simulink model "OptimalTracking_F16_Simulink"  (R2020b)
settings: Solver=VariableStepAuto  StartTime=0.0  StopTime=30  RelTol=1e-3
values from neighbouring files (symbols this model uses):
  A = [0 0 1 ... (first row only)    [OptimalTracking_F16.m]
  B = [0 ... (first row only)    [OptimalTracking_F16.m]
  C = [1 0 0]    [OptimalTracking_F16.m]
  G1 = -inv(C*inv(A-B*K1)*B)    [OptimalTracking_F16.m]
  G2 = -inv(C*inv(A-B*K2)*B)    [OptimalTracking_F16.m]
  G3 = -inv(C*inv(A-B*K3)*B)    [OptimalTracking_F16.m]
  G4 = -inv(C*inv(A-B*K4)*B)    [OptimalTracking_F16.m]
  G_f = -inv(C*inv(A-B*K_f)*B)    [OptimalTracking_F16.m]
  G_s = -inv(C*inv(A-B*K_s)*B)    [OptimalTracking_F16.m]
  G_t = -inv(C*inv(A-B*K_t)*B)    [OptimalTracking_F16.m]
  K1 = place(A,B,PO)    [OptimalTracking_F16.m]
  K2 = lqr(A,B,Q1,R1)    [OptimalTracking_F16.m]
  K3 = lqr(A,B,Q2,R2)    [OptimalTracking_F16.m]
  K4 = lqr(A,B,Q3,R3)    [OptimalTracking_F16.m]
  K_f = lqr(A,B,Q_u,r1)    [OptimalTracking_F16.m]
  K_s = lqr(A,B,Q_u,r2)    [OptimalTracking_F16.m]
  K_t = lqr(A,B,Q_u,r3)    [OptimalTracking_F16.m]
  u_opt = double(u_opt)    [Zermelo.m]
libraries: simulink_extras x6
settings Model: Creator=DELL  LastModifiedBy=DELL

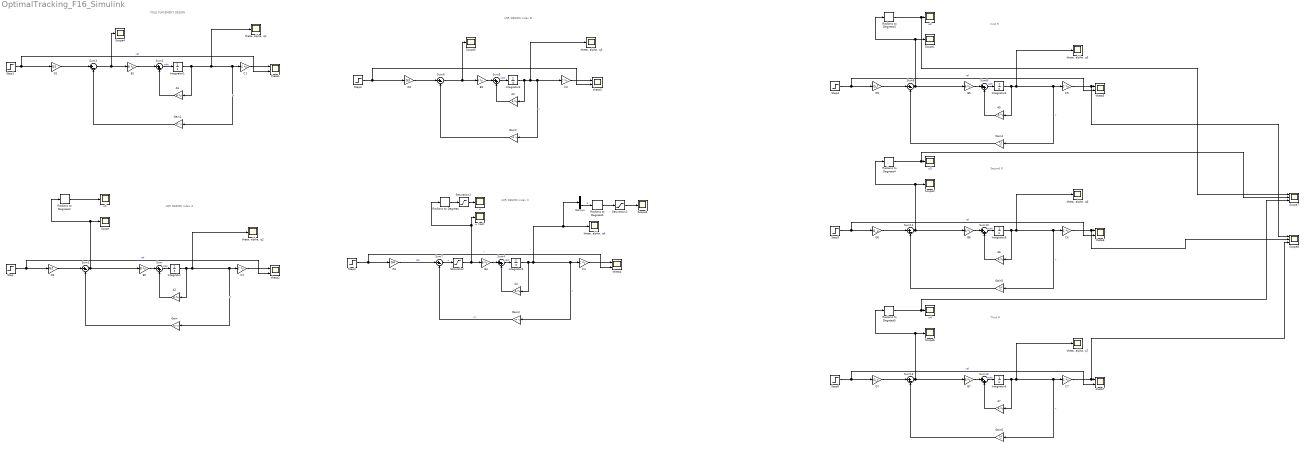
== system OptimalTracking_F16_Simulink ==
  note: LQR DESIGN
      | index A
  note: POLE PLACEMENT DESIGN
  note: LQR DESIGN
      | index B
  note: LQR DESIGN
      | index C
  note: First R
  note: Second R
  note: Third R
  A{1..7} (7 alike) : Gain  Gain=A  Multiplication=Matrix(K*u)
  B{1..7} (7 alike) : Gain  Gain=B  Multiplication=Matrix(K*u)
  C{1..7} (7 alike) : Gain  Gain=C  Multiplication=Matrix(K*u)
  Demux : Demux  Outputs=3
  G1 : Gain  Gain=G1
  G2 : Gain  Gain=G2
  G3 : Gain  Gain=G3
  G4 : Gain  Gain=G4
  G5 : Gain  Gain=G_f
  G6 : Gain  Gain=G_s
  G7 : Gain  Gain=G_t
  Gain : Gain  Gain=K2  Multiplication=Matrix(K*u)
  Gain1 : Gain  Gain=K1  Multiplication=Matrix(K*u)
  Gain2 : Gain  Gain=K3  Multiplication=Matrix(K*u)
  Gain3 : Gain  Gain=K4  Multiplication=Matrix(K*u)
  Gain4 : Gain  Gain=K_f  Multiplication=Matrix(K*u)
  Gain5 : Gain  Gain=K_s  Multiplication=Matrix(K*u)
  Gain6 : Gain  Gain=K_t  Multiplication=Matrix(K*u)
  Integrator{,1..6} (7 alike) : Integrator  InitialCondition=[0.046492 0.046492 0]'
  Radians to Degrees{,1..5} (6 alike) : simulink_extras/Transformations/Radians to Degrees
  Saturation : Saturate  UpperLimit=0.436332  LowerLimit=-0.436332
  Saturation1 : Saturate  UpperLimit=25  LowerLimit=-25
  Saturation2 : Saturate  UpperLimit=60  LowerLimit=-60
  Scope{,1..6} (7 alike) : Scope
  Scope7 : Scope  NumInputPorts=3
  Scope8 : Scope  NumInputPorts=3
  Step{,1..6} (7 alike) : Step  Time=0  After=u_opt  SampleTime=0
  Sum{,2,4..5,8,10,12} (7 alike) : Sum  Inputs=|++
  Sum{1,3,6..7,9,11,13} (7 alike) : Sum  Inputs=|+-
  theta, alpha, q{1..7} (7 alike) : Scope
  theta{1..7} (7 alike) : Scope  NumInputPorts=2
  u{,1..4} (5 alike) : Scope
  u (rad) : Scope
  wires:
  G2/1 -> Sum1/1
  Gain/1 -> Sum1/2
  Integrator/1 -> C2/1, Gain/1, "theta, alpha, q2"/1, A2/1  "x"
  G1/1 -> Sum3/1
  Gain1/1 -> Sum3/2
  B2/1 -> Sum/1
  Integrator1/1 -> C1/1, Gain1/1, "theta, alpha, q1"/1, A1/1  "x"
  C1/1 -> theta1/1
  B1/1 -> Sum2/1
  Sum3/1 -> Scope4/1, B1/1
  A2/1 -> Sum/2
  A1/1 -> Sum2/2
  C2/1 -> theta2/1
  Step/1 -> G2/1, theta2/2  "ref"
  Step1/1 -> G1/1, theta1/2  "ref"
  Sum2/1 -> Integrator1/1  "xdot"
  Sum/1 -> Integrator/1  "xdot"
  Sum5/1 -> Integrator2/1  "xdot"
  C3/1 -> theta3/1
  G3/1 -> Sum6/1
  Sum6/1 -> Scope5/1, B3/1
  B3/1 -> Sum5/1
  Integrator2/1 -> C3/1, Gain2/1, "theta, alpha, q3"/1, A3/1  "x"
  Step3/1 -> G3/1, theta3/2
  Gain2/1 -> Sum6/2
  A3/1 -> Sum5/2
  Gain3/1 -> Sum7/2  "Kx"
  C4/1 -> theta4/1
  B4/1 -> Sum4/1
  Radians to Degrees/1 -> Saturation1/1
  A4/1 -> Sum4/2
  Sum4/1 -> Integrator3/1  "xdot"
  Step2/1 -> G4/1, theta4/2  "r"
  Integrator3/1 -> C4/1, Gain3/1, Demux/1, "theta, alpha, q4"/1, A4/1  "x"
  Sum7/1 -> Saturation/1  "u"
  G4/1 -> Sum7/1  "G2r"
  Saturation/1 -> u (rad)/1, Radians to Degrees/1, B4/1
  Saturation1/1 -> u/1
  Demux/3 -> Radians to Degrees1/1  "q"
  Radians to Degrees1/1 -> Saturation2/1
  Saturation2/1 -> Scope3/1
  Radians to Degrees2/1 -> u1/1
  Sum1/1 -> B2/1, Radians to Degrees2/1, Scope/1
  Sum9/1 -> B5/1, Radians to Degrees3/1, Scope1/1
  B5/1 -> Sum8/1
  A5/1 -> Sum8/2
  Radians to Degrees3/1 -> Scope7/1, u2/1
  Integrator4/1 -> C5/1, Gain4/1, "theta, alpha, q5"/1, A5/1  "x"
  Sum8/1 -> Integrator4/1  "xdot"
  G5/1 -> Sum9/1
  Gain4/1 -> Sum9/2
  Step4/1 -> G5/1, theta5/2  "ref"
  C5/1 -> Scope8/1, theta5/1
  Sum11/1 -> B6/1, Radians to Degrees4/1, Scope2/1
  B6/1 -> Sum10/1
  A6/1 -> Sum10/2
  Radians to Degrees4/1 -> Scope7/2, u3/1
  Integrator5/1 -> C6/1, Gain5/1, "theta, alpha, q6"/1, A6/1  "x"
  Sum10/1 -> Integrator5/1  "xdot"
  G6/1 -> Sum11/1
  Gain5/1 -> Sum11/2
  Step5/1 -> G6/1, theta6/2  "ref"
  C6/1 -> Scope8/2, theta6/1
  Sum13/1 -> B7/1, Radians to Degrees5/1, Scope6/1
  B7/1 -> Sum12/1
  A7/1 -> Sum12/2
  Radians to Degrees5/1 -> Scope7/3, u4/1
  Integrator6/1 -> C7/1, Gain6/1, "theta, alpha, q7"/1, A7/1  "x"
  Sum12/1 -> Integrator6/1  "xdot"
  G7/1 -> Sum13/1
  Gain6/1 -> Sum13/2
  Step6/1 -> G7/1, theta7/2  "ref"
  C7/1 -> Scope8/3, theta7/1
